simulink library "Library"  (R2018a)
settings: Solver=VariableStepAuto  StartTime=0.0  StopTime=10.0  RelTol=1e-3
undefined symbols (not defined in the file or in its folder): Automatic_Test, Motor, Thermal
settings Model: Creator=PATILMP  LastModifiedBy=PATILMP

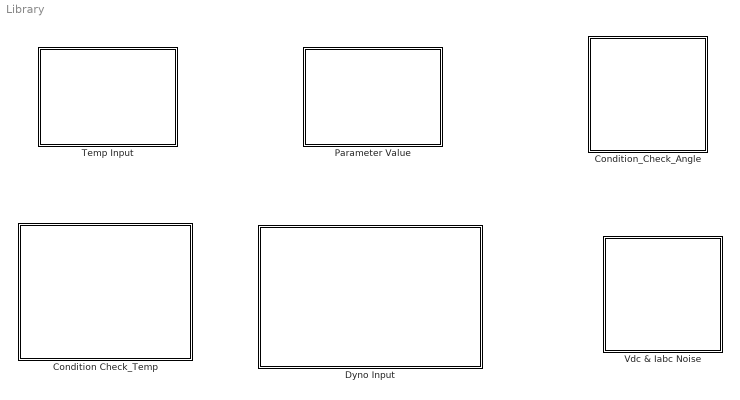
== system Library ==
  " Temp Input" : Subsystem
      mask Display: disp('Temperature Input')
  Condition Check_Temp : Subsystem
      mask Display: disp('Condition Check')
  Condition_Check_Angle : Subsystem  AncestorBlock=Library/Vdc & Iabc Noise
      mask Display: disp(' Condition_Check')
  Dyno Input : Subsystem
      mask Display: disp('Dyno Input')
  Parameter Value : Subsystem
      mask Display: disp('Parameter Value');
  Vdc & Iabc Noise : Subsystem
      mask Display: disp(' Vdc & Iabc Noise')

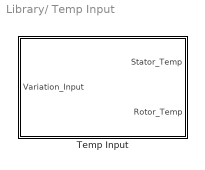
== system Library/ Temp Input ==
  Temp Input : MATLAB Function  TreatAsAtomicUnit=on  mask(Temp Input){Init_Value=Motor.Electrical.Rs_a_Ref, Temp_Ref=Motor.Mechanical.Rs_Temperature_Ref, alpha=Motor.Electrical.alpha_s, flag=strcmp(Automatic_Test.parameter_var,'Rs')}
      mask prompts: Init_Value "Parameter Intial Value"; Temp_Ref "Temperature Referance"; flag "Selection of Test"
      mask help: This Matlab function block is used to input temperature to stator and Rotor.

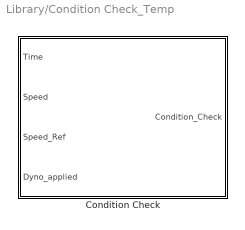
== system Library/Condition Check_Temp ==
  Condition Check : MATLAB Function  TreatAsAtomicUnit=on  mask(Condition Check){Speed_Tolerance=Automatic_Test.Speed_Tolerance, Para_time_check=Automatic_Test.Para_time_check}
      mask prompts: Speed_Tolerance "Speed Tolerance Value"; Para_time_check "Parameter Time Check"
      mask help: This function block keeps check on failurity of the Test.

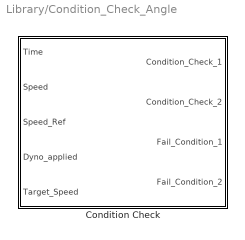
== system Library/Condition_Check_Angle ==
  Condition Check : MATLAB Function  TreatAsAtomicUnit=on  mask(ConditionCheck){Speed_Tolerance=Automatic_Test.Speed_Tolerance, Para_time_check_1=Automatic_Test.Para_time_check_1, Para_time_check_2=Automatic_Test.Para_time_check_2, Para_time_check_3=Automatic_Test.Para_time_check_3, Speed_Tolerance_1=Automatic_Test.Speed_Tolerance_1}
      mask prompts: Speed_Tolerance "Speed Tolerance Value"; Para_time_check_1 "Prameter Time Check_1"; Para_time_check_2 "Para_Time_Check"; Speed_Tolerance_1 "Speed Tolerance Value_1"
      mask help: This block is used to check failure conditions.

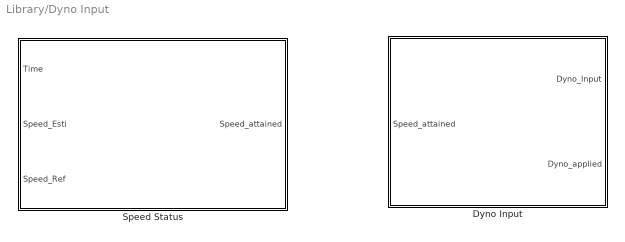
== system Library/Dyno Input ==
  Dyno Input : MATLAB Function  TreatAsAtomicUnit=on  mask(Dyno Input){Dyno_Load=Automatic_Test.Dyno_Load, Dyno_Step_Size=Automatic_Test.Dyno_Step_Size}
      mask prompts: Dyno_Load "Dyno Load Value"; Dyno_Step_Size "Dyno Step Size"
      mask help: This Matlab function block is used to input Dyno load.
  Speed Status : MATLAB Function  TreatAsAtomicUnit=on  mask(Speed Status){Status_Tolerance=Automatic_Test.Status_Tolerance, Status_Time_Check=Automatic_Test.Status_Time_Check}
      mask prompts: Status_Tolerance "Status Tolerance"; Status_Time_Check "Status Time Check"
      mask help: This Matlab function block is used to get the status of reference and estimated speed.

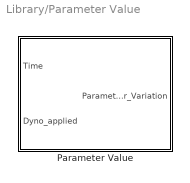
== system Library/Parameter Value ==
  Parameter Value : MATLAB Function  TreatAsAtomicUnit=on  mask(Parameter value){init_value=Motor.Electrical.Rs_a_Ref, Para_time_check=Automatic_Test.Para_time_check, Percentage_Variation=Automatic_Test.Percentage_Variation}
      mask prompts: init_value "Intital Value"; Para_time_check "Time_Check"; Percentage_Variation "Percentage Variation"
      mask help: This Matlab function block is used to input the parameter variation signal.

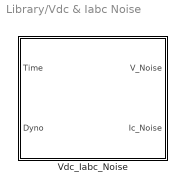
== system Library/Vdc & Iabc Noise ==
  Vdc_Iabc_Noise : Subsystem  mask(Vdc_Iabc_Noise){}
      mask help: This block is used to impose noise on Vdc and Iabc inputs.
      mask Help: web('Vdc_Iabc_Noise.htm')
      mask Display:
      | port_label('Input',1,'Time');
      | port_label('Input',2,'Dyno_Input');
      | port_label('Output',1,'V_Noise');
      | port_label('Output',2,'Ic_Noise');

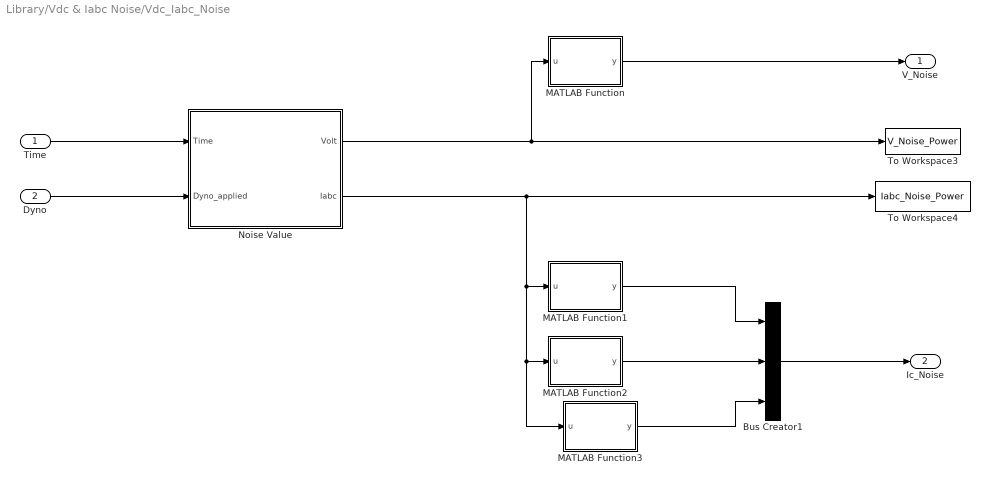
== system Library/Vdc & Iabc Noise/Vdc_Iabc_Noise ==
  Time : Inport
  Dyno : Inport  Port=2
  Bus Creator1 : BusCreator  Inputs=3
  MATLAB Function : MATLAB Function  TreatAsAtomicUnit=on
  MATLAB Function1 : MATLAB Function  TreatAsAtomicUnit=on
  MATLAB Function2 : MATLAB Function  TreatAsAtomicUnit=on
  MATLAB Function3 : MATLAB Function  TreatAsAtomicUnit=on
  Noise Value : MATLAB Function  TreatAsAtomicUnit=on  mask(Parameter Value){init_value=Automatic_Test.Volt, Para_time_check=Automatic_Test.Status_Time_Check, Percentage_Variation=Automatic_Test.Percentage_Variation_Noise, flag=strcmp(Automatic_Test.Noise_Var,'Volt_Noise_Power')}
      mask prompts: init_value "Intital Value"; Para_time_check "Time_Check"; Percentage_Variation "Percentage Variation"; flag "Selection of test"
      mask help: This Matlab function block is used to input the parameter variation signal.
  To Workspace3 : ToWorkspace  VariableName=V_Noise_Power  SaveFormat=Structure  SampleTime=-1
  To Workspace4 : ToWorkspace  VariableName=Iabc_Noise_Power  SaveFormat=Structure  SampleTime=-1
  V_Noise : Outport
  Ic_Noise : Outport  Port=2
  wires:
  Time/1 -> Noise Value/1(Time)
  Dyno/1 -> Noise Value/2(Dyno_applied)
  Noise Value/1(Volt) -> MATLAB Function/1(u), To Workspace3/1
  MATLAB Function/1(y) -> V_Noise/1
  MATLAB Function1/1(y) -> Bus Creator1/1
  MATLAB Function2/1(y) -> Bus Creator1/2
  MATLAB Function3/1(y) -> Bus Creator1/3
  Bus Creator1/1 -> Ic_Noise/1
  Noise Value/2(Iabc) -> To Workspace4/1, MATLAB Function3/1(u), MATLAB Function2/1(u), MATLAB Function1/1(u)

== matlab function Library/Parameter Value/Parameter Value ==
  data: Time input; Dyno_applied input; Parameter_Variation output; Para_time_check parameter; Percentage_Variation parameter; init_value parameter

function Parameter_Variation   = fcn(Time,Dyno_applied,Para_time_check, Percentage_Variation,init_value)
persistent old_value
persistent old_time
% step=Percentage/100;  % later put as parameter



step=(Percentage_Variation/100)*init_value;


if isempty(old_value)
    old_value=init_value;
end
   
if isempty(old_time)
    old_time=0;
end

if Dyno_applied==1
    if ((Time-old_time)> Para_time_check)
        old_time=Time;
        old_value= old_value+step;
       
    end
    
else
    old_time=Time;
end
    

Parameter_Variation =old_value;

== matlab function Library/Condition Check_Temp/Condition Check ==
  data: Time input; Speed input; Speed_Ref input; Condition_Check output; Dyno_applied input; Speed_Tolerance parameter; Para_time_check parameter
function Condition_Check = fcn(Time,Speed,Speed_Ref,Dyno_applied, Speed_Tolerance,Para_time_check)
persistent old_value
if isempty(old_value)
    old_value=0;
end

ST=Speed_Tolerance/100;
Limit=Speed_Ref*ST;
Delta_Speed=abs(Speed-Speed_Ref);


Condition_Check = 0;

if Dyno_applied==1
    if (Delta_Speed > Limit)
        if ((Time-old_value)>0.3*Para_time_check)
            Condition_Check = 1; 
        end
    else
        old_value = Time;
    end
end

== matlab function Library/Condition_Check_Angle/Condition Check ==
  data: Condition_Check_1 output; Condition_Check_2 output; Fail_Condition_1 output; Time input; Speed input; Speed_Ref input; Dyno_applied input; Speed_Tolerance parameter; Para_time_check_1 parameter; Para_time_check_2 parameter; Para_time_check_3 parameter; Speed_Tolerance_1 parameter; Target_Speed input; Fail_Condition_2 output
function [Condition_Check_1,Condition_Check_2,Fail_Condition_1,Fail_Condition_2] = fcn(Time,Speed,Speed_Ref,Dyno_applied,Speed_Tolerance,Para_time_check_1,Para_time_check_2,Para_time_check_3,Speed_Tolerance_1,Target_Speed)

persistent old_value1
persistent old_value2
persistent old_value3
persistent count

if isempty(old_value1)
    old_value1=0;
end
if isempty(old_value2)
    old_value2=0;
end
if isempty(old_value3)
    old_value3=0;
end

if isempty(count)
    count=0;
end

ST=Speed_Tolerance/100;
ST1=Speed_Tolerance_1/100;
Limit=Speed_Ref*ST;
Delta_Speed=abs(Speed-Speed_Ref);

Fail_Condition_1=0;
Fail_Condition_2=0;
Condition_Check_1 = 0;
Condition_Check_2 = 0;

%if Dyno_applied==1
 if (Delta_Speed > Limit)
        if((Time-old_value1)>Para_time_check_2)
             Fail_Condition_1= 1;  
        elseif((Time-old_value2)>Para_time_check_1)
            count = count+1;
            old_value2 = Time; 
         end
 else
        old_value1 = Time;
 end 
%end

 if int32(Speed_Ref) >= Target_Speed
     old_value3 = Time;
     if (Speed>= Speed_Ref+ST1*Speed_Ref)
    if(old_value3> Para_time_check_3)
    Fail_Condition_2= 1;
    end
     end
if count > 1
    Condition_Check_2 = 1; 
elseif(count==1)
    Condition_Check_1 = 1; 
else
Condition_Check_1 = 0;
Condition_Check_2 = 0;
    
end

end







%      old_value1=Time;
%  
% if (Speed>= Speed_Ref+ST1*Speed_Ref && Time)
%     if(old_value1> Para_time_check_3)
%     Fail_Condition_2= 1;
%     end
% end








% function [Condition_Check_1,Condition_Check_2,Fail_Condition_1,Fail_Condition_2,Delta_Speed,Limit] = fcn(Time,Speed,Speed_Ref,Dyno_applied,Target_Speed,Speed_Tolerance,Para_time_check_1,Para_time_check_2,Para_time_check_3,Speed_Tolerance_1)
% 
% persistent old_value
% persistent old_value1
% persistent count
% 
% if isempty(old_value)
%     old_value=0;
% end
% if isempty(old_value1)
%     old_value1=0;
% end
% 
% if isempty(count)
%     count=0;
% end
% 
% ST=Speed_Tolerance/100;
% ST1=Speed_Tolerance_1/100;
% Limit=Speed_Ref+Speed_Ref*ST;
% Delta_Speed=abs(Speed);%-Speed_Ref);
% 
% Fail_Condition_1=0;
% Fail_Condition_2=0;
% Condition_Check_1 = 0;
% Condition_Check_2 = 0;
% 
%  if (Delta_Speed > Limit)
%   count = count+1;
%   else
%         old_value = Time;
%  end 
% 
% if Speed_Ref >= Target_Speed
% if count > 1
%     Condition_Check_2 = 1; 
% elseif(count==1)
%     Condition_Check_1 = 1; 
% else
% Condition_Check_1 = 0;
% Condition_Check_2 = 0;
%     
% end
% 
% end
% 
% 
% 
% 



%      old_value1=Time;
%  
% if (Speed>= Speed_Ref+ST1*Speed_Ref && Time)
%     if(old_value1> Para_time_check_3)
%     Fail_Condition_2= 1;
%     end
% end






% if Speed_Ref >= Target_Speed
%     
% if count > 1
%     Condition_Check_2 = 1; 
% elseif(count==1)
%     Condition_Check_1 = 1; 
% else
% Condition_Check_1 = 0;
% Condition_Check_2 = 0;
%     
% end
% 
% end
% 
% function [Condition_Check_1,Condition_Check_2,Fail_Condition_1,Fail_Condition_2] = fcn(Time,Speed,Speed_Ref,Dyno_applied,Target_Speed,Speed_Tolerance,Para_time_check_1,Para_time_check_2,Para_time_check_3,Speed_Tolerance_1)
% 
% persistent old_value
% persistent old_value1
% persistent count
% 
% if isempty(old_value)
%     old_value=0;
% end
% if isempty(old_value1)
%     old_value1=0;
% end
% 
% if isempty(count)
%     count=0;
% end
% 
% ST=Speed_Tolerance/100;
% ST1=Speed_Tolerance_1/100;
% Limit=Speed_Ref*ST;
% Delta_Speed=abs(Speed-Speed_Ref);
% 
% Fail_Condition_1=0;
% Fail_Condition_2=0;
% Condition_Check_1 = 0;
% Condition_Check_2 = 0;
% 
% if Dyno_applied==1
%  if (Delta_Speed > Limit)
%         if((Time-old_value)>Para_time_check_2)
%              Fail_Condition_1= 1;  
%         elseif((Time-old_value)>Para_time_check_1)
%             count = count+1;
%               old_value = Time;
%          end
%  else
%         old_value = Time;
%  end 
% end
% 
% if Speed_Ref >= Target_Speed
% 
% if count > 1
%     Condition_Check_2 = 1; 
% elseif(count==1)
%     Condition_Check_1 = 1; 
% else
% Condition_Check_1 = 0;
% Condition_Check_2 = 0;
%     
% end
% 
% end
% 
% 
% 
% 
% 
% 
% 
% %      old_value1=Time;
% %  
% % if (Speed>= Speed_Ref+ST1*Speed_Ref && Time)
% %     if(old_value1> Para_time_check_3)
% %     Fail_Condition_2= 1;
% %     end
% % end
% 
% 
% 
% 
% 
% 0
% % if Speed_Ref >= Target_Speed
% %     
% % if count > 1
% %     Condition_Check_2 = 1; 
% % elseif(count==1)
% %     Condition_Check_1 = 1; 
% % else
% % Condition_Check_1 = 0;
% % Condition_Check_2 = 0;
% %     
% % end
% % 
% % end
% % 
% 
%

== matlab function Library/Dyno Input/Dyno Input ==
  data: Dyno_Input output; Speed_attained input; Dyno_applied output; Dyno_Load parameter; Dyno_Step_Size parameter
function [Dyno_Input,Dyno_applied] = fcn(Speed_attained, Dyno_Load,Dyno_Step_Size )
persistent old_value
 


init_value=0;
Dyno_applied=0;

if isempty(old_value)
    old_value=init_value;
    
end

if Speed_attained==1
    old_value=Dyno_Step_Size+old_value;
    
     if old_value>Dyno_Load
         
         old_value=Dyno_Load;
         Dyno_applied=1;
    end 
end

Dyno_Input=old_value;

== matlab function Library/Vdc & Iabc Noise/Vdc_Iabc_Noise/MATLAB Function ==
  data: u input; y output
function y = fcn(u)
y =0 + sqrt(u) * randn(1,1);

== matlab function Library/Vdc & Iabc Noise/Vdc_Iabc_Noise/MATLAB Function1 ==
  data: u input; y output
function y = fcn(u)
y =0 + sqrt(u) * randn(1,1);

== matlab function Library/Vdc & Iabc Noise/Vdc_Iabc_Noise/MATLAB Function2 ==
  data: u input; y output
function y = fcn(u)
y =0 + sqrt(u) * randn(1,1);

== matlab function Library/Vdc & Iabc Noise/Vdc_Iabc_Noise/MATLAB Function3 ==
  data: u input; y output
function y = fcn(u)
y =0 + sqrt(u) * randn(1,1);

== matlab function Library/Vdc & Iabc Noise/Vdc_Iabc_Noise/Noise Value ==
  data: Time input; Dyno_applied input; Volt output; Para_time_check parameter; Percentage_Variation parameter; init_value parameter; Iabc output; flag parameter

function [Volt,Iabc]= fcn(Time,Dyno_applied,Para_time_check,Percentage_Variation,init_value,flag)
persistent old_value
persistent old_time

Volt=0;
Iabc=0;

step=(Percentage_Variation/100)*init_value;


if isempty(old_value)
    old_value=init_value;
end
   
if isempty(old_time)
    old_time=0;
end

if Dyno_applied==1
    if ((Time-old_time)> Para_time_check)
        old_time=Time;
        old_value= old_value+step;
       
    end
    
else
    old_time=Time;
end


if(flag==1)
Volt=old_value; 
Iabc=0;
end
if(flag==0)
Iabc=old_value; 
 Volt=0;
end

== matlab function Library/ Temp Input/Temp Input ==
  data: Variation_Input input; Init_Value parameter; Temp_Ref parameter; Stator_Temp output; alpha parameter; Thermal parameter; Rotor_Temp output; flag parameter
function [Stator_Temp,Rotor_Temp] = fcn(Variation_Input,Init_Value,Temp_Ref,alpha,Thermal,flag) %fcn(Input,Init_Value, Temp_Ref,alpha)
Stator_Temp=0;
Rotor_Temp=0;
%......Calculation of Temperature T with corrosponding change in Parameter....%

 Temp=(Variation_Input+Init_Value*(alpha*Temp_Ref-1))/(Init_Value*alpha);
 
if(flag==1)
Stator_Temp=Temp; 
Rotor_Temp= Thermal.Trotor;
 end
if(flag==0)
 Rotor_Temp=Temp; 
 Stator_Temp=Thermal.Tstator;
end









% 
% function [Stator_Temp,Rotor_Temp] = fcn(Input,Init_Value,Temp_Ref,alpha,Thermal,flag) %fcn(Input,Init_Value, Temp_Ref,alpha)
% Stator_Temp=0;
% Rotor_Temp=0;
% %......Calculation of Temperature T with corrosponding change in Parameter....%
% 
%  Temp=(Input+Init_Value*(alpha*Temp_Ref-1))/(Init_Value*alpha);
%  
% if(flag==1)
% Stator_Temp=Temp; 
% Rotor_Temp= Thermal.Trotor;
%  end
% if(flag==0)
%  Rotor_Temp=Temp; 
%  Stator_Temp=Thermal.Tstator;
% end

== matlab function Library/Dyno Input/Speed Status ==
  data: Speed_attained output; Time input; Speed_Esti input; Speed_Ref input; Status_Tolerance parameter; Status_Time_Check parameter
function Speed_attained = fcn(Time,Speed_Esti,Speed_Ref,Status_Tolerance,Status_Time_Check)
persistent t_old
persistent flag


if isempty(t_old)
    t_old =0;
end

if isempty(flag)
    flag = 0;
end

if abs(Speed_Ref- Speed_Esti)<(Status_Tolerance*Speed_Ref)
   flag = 1;
end

if flag == 0
    t_old = Time;
end

if (Time-t_old)>Status_Time_Check
    Speed_attained = 1;
else
    Speed_attained = 0;
end
